simulink model "Counter"  (R2025a)
settings: Solver=FixedStepAuto  StartTime=0.0  StopTime=2  FixedStep=0.1  RelTol=1e-3
settings Model: Creator=Shailesh Jaiswal  LastModifiedBy=Shailesh Jaiswal

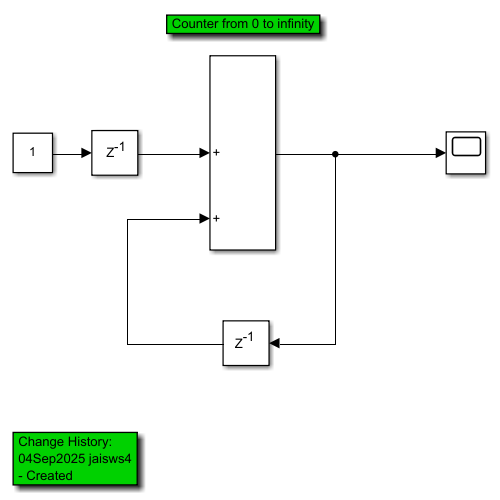
[thumbnail: Simulink's stored preview of the top-level diagram]
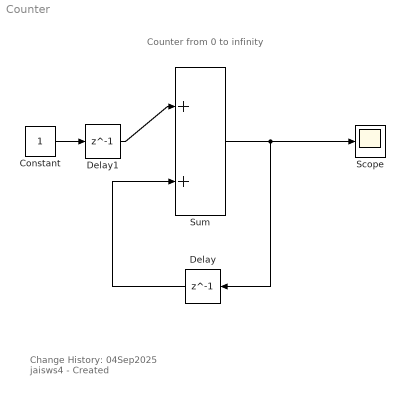
== system Counter ==
  note: Counter from 0 to infinity
  note: Change History:
      | 04Sep2025 jaisws4
      | - Created
  Constant : Constant
  Delay : Delay  DelayLength=1
  Delay1 : Delay  DelayLength=1
  Scope : Scope
      settings: ActiveDisplayYMinimum=-2.4999999999999996  ActiveDisplayYMaximum=22.5
  Sum : Sum  Inputs=|++
  wires:
  Constant/1 -> Delay1/1
  Delay/1 -> Sum/2
  Sum/1 -> Scope/1, Delay/1
  Delay1/1 -> Sum/1
